simulink model "Lesson_1_model"  (R2022b)
settings: Solver=VariableStepAuto  StartTime=0.0  StopTime=100.0  RelTol=1e-3
values from neighbouring files (symbols this model uses):
  A1 = expm(A*dt1)    [Lecture1_1.m]
  A2 = expm(A*dt2)    [Lecture1_1.m]
  A3 = expm(A*dt3)    [Lecture1_1.m]
  B1 = inv(A) * (A1 - eye(size(A))) * B    [Lecture1_1.m]
  B2 = inv(A) * (A2 - eye(size(A))) * B    [Lecture1_1.m]
  B3 = inv(A) * (A3 - eye(size(A))) * B    [Lecture1_1.m]
  C = [1 0 1]    [Lecture1_1.m]
  dt1 = 0.2    [Lecture1_1.m]
  dt2 = 0.033    [Lecture1_1.m]
  dt3 = 0.01    [Lecture1_1.m]
  GpssConA = GpssObsA.'    [Lecture_1.m]
  GpssConA1 = expm(GpssConA*dt1)    [Lecture_1.m]
  GpssConA2 = expm(GpssConA*dt2)    [Lecture_1.m]
  GpssConA3 = expm(GpssConA*dt3)    [Lecture_1.m]
  GpssConB = GpssObsC.'    [Lecture_1.m]
  GpssConB1 = inv(GpssConA) * (GpssConA1 - eye(size(GpssConA))) * GpssConB    [Lecture_1.m]
  GpssConB2 = inv(GpssConA) * (GpssConA2 - eye(size(GpssConA))) * GpssConB    [Lecture_1.m]
  GpssConB3 = inv(GpssConA) * (GpssConA3 - eye(size(GpssConA))) * GpssConB    [Lecture_1.m]
  GpssConC = GpssObsB.'    [Lecture_1.m]
  GpssConD = GpssObsD    [Lecture_1.m]
  GpssObsA = GpssObs.A    [Lecture_1.m]
  GpssObsB = GpssObs.B    [Lecture_1.m]
  GpssObsC = GpssObs.C    [Lecture_1.m]
  GpssObsD = GpssObs.D    [Lecture_1.m]
settings Model: Creator=ilya  LastModifiedBy=ilya

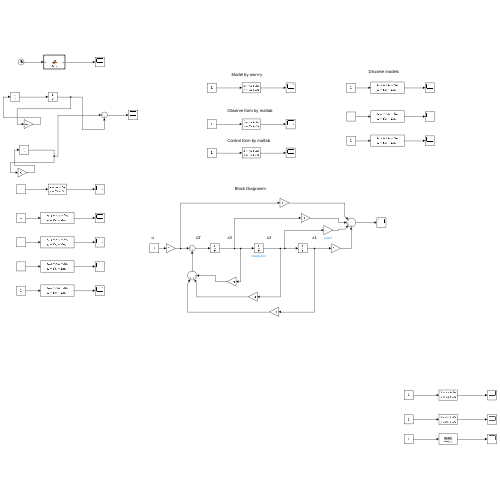
[thumbnail: Simulink's stored preview of the top-level diagram]
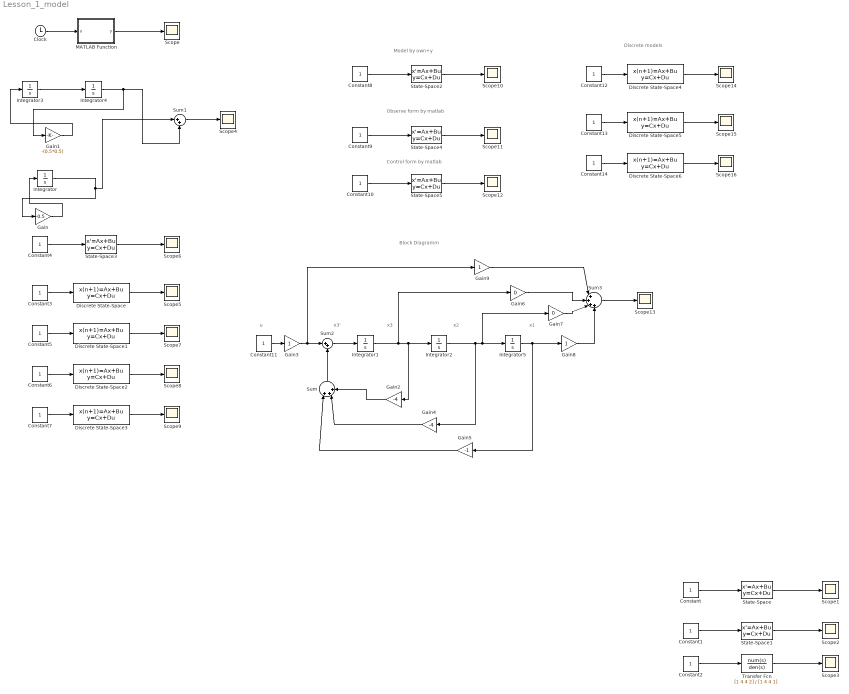
== system Lesson_1_model ==
  note: Model by own+y
  note: Observe form by matlab
  note: Control form by matlab
  note: Block Diagramm
  note: x1
  note: x2
  note: x3
  note: x3'
  note: u
  note: Discrete models
  Clock : Clock
  Constant{,1..14} (15 alike) : Constant
  Discrete State-Space : DiscreteStateSpace  A="[ 0.9950  0.1997  0; -0.0499  0.9950   0;  0  0  0.9048]"  B=[0; 0; 0]  C=[1 0 1]  D=0  InitialCondition=[1; 0; 1]  SampleTime=0.2
  Discrete State-Space1 : DiscreteStateSpace  A=A1  B=B1  C=C  D=0  InitialCondition=[1; 0; 1]  SampleTime=dt1
  Discrete State-Space2 : DiscreteStateSpace  A=A2  B=B2  C=C  D=0  InitialCondition=[1; 0; 1]  SampleTime=dt2
  Discrete State-Space3 : DiscreteStateSpace  A=A3  B=B3  C=C  D=0  InitialCondition=[1; 0; 1]  SampleTime=dt3
  Discrete State-Space4 : DiscreteStateSpace  A=GpssConA1  B=GpssConB1  C=GpssConC  D=GpssConD  SampleTime=dt1
  Discrete State-Space5 : DiscreteStateSpace  A=GpssConA2  B=GpssConB2  C=GpssConC  D=GpssConD  SampleTime=dt2
  Discrete State-Space6 : DiscreteStateSpace  A=GpssConA3  B=GpssConB3  C=GpssConC  D=GpssConD  SampleTime=dt3
  Gain : Gain  Gain=-0.5
  Gain1 : Gain  Gain=-(0.5*0.5)
  Gain2 : Gain  Gain=-4
  Gain3 : Gain
  Gain4 : Gain  Gain=-4
  Gain5 : Gain  Gain=-1
  Gain6 : Gain  Gain=0
  Gain7 : Gain  Gain=0
  Gain8 : Gain
  Gain9 : Gain
  Integrator : Integrator  InitialCondition=1
  Integrator{1..3,5} (4 alike) : Integrator
  Integrator4 : Integrator  InitialCondition=1
  MATLAB Function : MATLAB Function  TreatAsAtomicUnit=on
  Scope{,1..16} (17 alike) : Scope
  State-Space : StateSpace  A=[0 1 0 0; 0 0 1 0; 0 0 0 1 ; -1 -4 -4 -1]  B=[0; 0; 0; 1]  C=[2 4 4 1]  D=0  InitialCondition=0
  State-Space1 : StateSpace  A=[0 1 0; 0 0 1; -1 -4 -4]  B=[0; 0; 1]  C=[1 0 0]  D=0  InitialCondition=0
  State-Space2 : StateSpace  A=[0 1 0; 0 0 1; -1 -4 -4]  B=[0; 0; 1]  C=[1 0 0]  InitialCondition=0
  State-Space3 : StateSpace  A=[0 1 0; -0.25 0 0; 0 0 -0.5]  B=[0; 0; 0]  C=[1 0 1]  D=0  InitialCondition=[1; 0; 1]
  State-Space4 : StateSpace  A=GpssObsA  B=GpssObsB  C=GpssObsC  D=GpssObsD  InitialCondition=0
  State-Space5 : StateSpace  A=GpssConA  B=GpssConB  C=GpssConC  D=GpssConD  InitialCondition=0
  Sum : Sum  Inputs=|+++
  Sum1 : Sum  Inputs=|++
  Sum2 : Sum  Inputs=|++
  Sum3 : Sum  Inputs=|++++
  Transfer Fcn : TransferFcn  Numerator=[1 4 4 2]  Denominator=[1 4 4 1]
  wires:
  Clock/1 -> MATLAB Function/1(u)
  MATLAB Function/1(y) -> Scope/1
  State-Space/1 -> Scope1/1
  Constant/1 -> State-Space/1
  State-Space1/1 -> Scope2/1
  Constant1/1 -> State-Space1/1
  Transfer Fcn/1 -> Scope3/1
  Constant2/1 -> Transfer Fcn/1
  Gain/1 -> Integrator/1
  Integrator/1 -> Sum1/1, Gain/1
  Integrator3/1 -> Integrator4/1
  Integrator4/1 -> Sum1/2, Gain1/1
  Gain1/1 -> Integrator3/1
  Sum1/1 -> Scope4/1
  Constant4/1 -> State-Space3/1
  State-Space3/1 -> Scope6/1
  Discrete State-Space/1 -> Scope5/1
  Constant3/1 -> Discrete State-Space/1
  Constant5/1 -> Discrete State-Space1/1
  Discrete State-Space1/1 -> Scope7/1
  Discrete State-Space2/1 -> Scope8/1
  Constant6/1 -> Discrete State-Space2/1
  Constant7/1 -> Discrete State-Space3/1
  Discrete State-Space3/1 -> Scope9/1
  State-Space2/1 -> Scope10/1
  Constant8/1 -> State-Space2/1
  Constant9/1 -> State-Space4/1
  State-Space4/1 -> Scope11/1
  State-Space5/1 -> Scope12/1
  Constant10/1 -> State-Space5/1
  Integrator2/1 -> Gain7/1, Integrator5/1, Gain4/1
  Integrator1/1 -> Gain6/1, Gain2/1, Integrator2/1
  Integrator5/1 -> Gain8/1, Gain5/1
  Gain2/1 -> Sum/3
  Gain4/1 -> Sum/2
  Gain5/1 -> Sum/1
  Constant11/1 -> Gain3/1
  Sum/1 -> Sum2/2
  Gain3/1 -> Gain9/1, Sum2/1
  Sum2/1 -> Integrator1/1
  Gain8/1 -> Sum3/4
  Gain7/1 -> Sum3/3
  Gain6/1 -> Sum3/2
  Gain9/1 -> Sum3/1
  Sum3/1 -> Scope13/1
  Constant12/1 -> Discrete State-Space4/1
  Discrete State-Space4/1 -> Scope14/1
  Discrete State-Space5/1 -> Scope15/1
  Constant13/1 -> Discrete State-Space5/1
  Constant14/1 -> Discrete State-Space6/1
  Discrete State-Space6/1 -> Scope16/1

== matlab function Lesson_1_model/MATLAB Function ==
  data: u input; y output
function y = fcn(u)

y = exp(-0.5*u) + cos(-0.5 * u);
